simulink model "sis_caotico"  (Simulink 7.7)
settings: Solver=ode45  StartTime=0.0  StopTime=10  RelTol=1e-6
values from neighbouring files (symbols this model uses):
  g = 10    [Ex3.m]    (also in Ex34.m)
  l = 1    [Ex3.m]    (also in Ex34.m)
  m = 50    [Ex3.m]    (also in Ex34.m)
  p10 = 0    [Ex3.m]    (also in Ex34.m)
  p20 = 0    [Ex3.m]    (also in Ex34.m)
  teta10 = 25*pi/180    (= 0.436332312999)    [Ex3.m]
  teta20 = 25*pi/180    (= 0.436332312999)    [Ex3.m]
settings Model: Creator=g  LastModifiedBy=g
settings DebuggingCC: SolverPrmCheckMsg=none

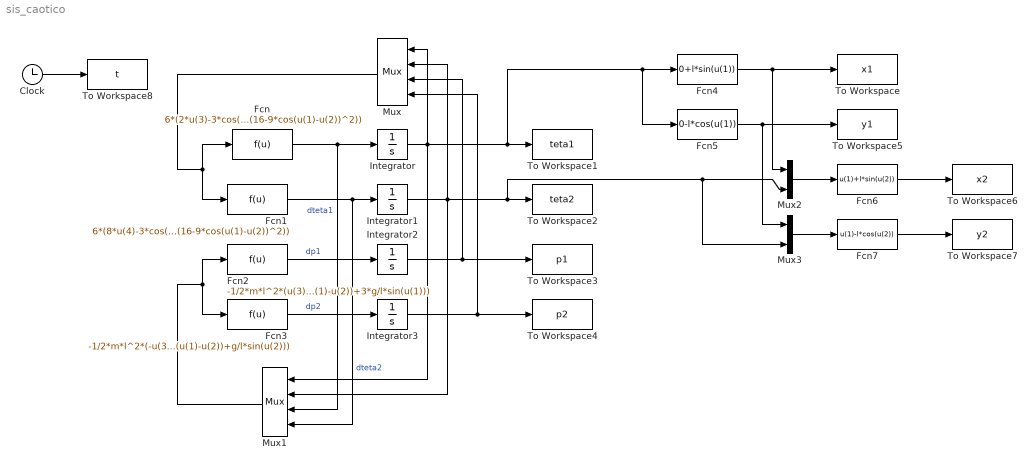
== system sis_caotico ==
  Clock : Clock
      settings: Decimation=10
  Fcn : Fcn  Expr=6*(2*u(3)-3*cos(u(1)-u(2))*u(4))/((m*l^2)*(16-9*cos(u(1)-u(2))^2))
  Fcn1 : Fcn  Expr=6*(8*u(4)-3*cos(u(1)-u(2))*u(3))/((m*l^2)*(16-9*cos(u(1)-u(2))^2))
  Fcn2 : Fcn  Expr=-1/2*m*l^2*(u(3)*u(4)*sin(u(1)-u(2))+3*g/l*sin(u(1)))
  Fcn3 : Fcn  Expr=-1/2*m*l^2*(-u(3)*u(4)*sin(u(1)-u(2))+g/l*sin(u(2)))
  Fcn4 : Fcn  Expr=0+l*sin(u(1))
  Fcn5 : Fcn  Expr=0-l*cos(u(1))
  Fcn6 : Fcn  Expr=u(1)+l*sin(u(2))
  Fcn7 : Fcn  Expr=u(1)-l*cos(u(2))
  Integrator : Integrator  InitialCondition=teta10
  Integrator1 : Integrator  InitialCondition=teta20
  Integrator2 : Integrator  InitialCondition=p10
  Integrator3 : Integrator  InitialCondition=p20
  Mux : Mux
  Mux1 : Mux
  Mux2 : Mux  Inputs=2
  Mux3 : Mux  Inputs=2
  To Workspace : ToWorkspace  VariableName=x1  SampleTime=-1  SaveFormat=Array
  To Workspace1 : ToWorkspace  VariableName=teta1  SampleTime=-1  SaveFormat=Array
  To Workspace2 : ToWorkspace  VariableName=teta2  SampleTime=-1  SaveFormat=Array
  To Workspace3 : ToWorkspace  VariableName=p1  SampleTime=-1  SaveFormat=Array
  To Workspace4 : ToWorkspace  VariableName=p2  SampleTime=-1  SaveFormat=Array
  To Workspace5 : ToWorkspace  VariableName=y1  SampleTime=-1  SaveFormat=Array
  To Workspace6 : ToWorkspace  VariableName=x2  SampleTime=-1  SaveFormat=Array
  To Workspace7 : ToWorkspace  VariableName=y2  SampleTime=-1  SaveFormat=Array
  To Workspace8 : ToWorkspace  VariableName=t  SampleTime=-1  SaveFormat=Array
  wires:
  Integrator/1 -> Mux/1, Mux1/1, To Workspace1/1, Fcn4/1, Fcn5/1
  Fcn/1 -> Integrator/1, Mux1/3  "dteta1"
  Mux/1 -> Fcn/1, Fcn1/1
  Fcn1/1 -> Integrator1/1, Mux1/4  "dteta2"
  Fcn2/1 -> Integrator2/1  "dp1"
  Fcn3/1 -> Integrator3/1  "dp2"
  Integrator1/1 -> Mux/2, Mux1/2, To Workspace2/1, Mux2/2, Mux3/2
  Integrator2/1 -> To Workspace3/1, Mux/3
  Integrator3/1 -> To Workspace4/1, Mux/4
  Mux1/1 -> Fcn2/1, Fcn3/1
  Clock/1 -> To Workspace8/1
  Fcn4/1 -> Mux2/1, To Workspace/1
  Fcn5/1 -> Mux3/1, To Workspace5/1
  Fcn6/1 -> To Workspace6/1
  Fcn7/1 -> To Workspace7/1
  Mux2/1 -> Fcn6/1
  Mux3/1 -> Fcn7/1
